simulink library "lib_wheel2"  (Simulink 10.1)
settings: Solver=VariableStepAuto  StartTime=0.0  StopTime=10.0  RelTol=1e-3
undefined symbols (not defined in the file or in its folder): lib_help, NOTES, veh_air_density, veh_CD, veh_cg_height, veh_FA, veh_front_wt_frac, veh_gravity, veh_roadwheel_radius, veh_rr_a, veh_rr_alpha, veh_rr_b, veh_rr_beta, veh_rr_c, veh_wheelbase, wh_1st_rrc, wh_2nd_rrc, wh_axle_loss_mass, wh_axle_loss_trq, wh_fa_dl_brake_frac, wh_fa_dl_brake_mph, wh_fa_fric_brake_frac, wh_fa_fric_brake_mph, wh_front_active_bool, wh_inertia, wh_max_front_brake_force, wh_max_rear_brake_force, wh_pressure, wh_radius, wh_rear_active_bool, wh_slip, wh_slip_force_coeff
undefined symbols (not defined in the file): logFlag
libraries: $bdroot x61, lib_vehicle x2, lib_etc x2, lib_controls x2, lib_wheel x1
(part 2 of 13)

== system lib_wheel2/Submodels/front and rear brake controller (achievable)/braking force supplied by front friction brakes (N) ==
  add'l braking force req'd (N) : Inport
  possible speed (mph) : Inport  Port=2
  max front brake force (N) : Inport  Port=3
  Block NOTES : Subsystem
      mask Display: disp('Block\nNOTES')
  Constant : Constant  Value=1+eps
  Constant1 : Constant  Value=0.6
  Keep 0<frac<1 : Saturate  UpperLimit=1  LowerLimit=0
  MinMax : MinMax  Function=max  Inputs=2
  Product : Product  Inputs=**  SaturateOnIntegerOverflow=on
  Product1 : Product  Inputs=*/  SaturateOnIntegerOverflow=on
  Saturation : Saturate  UpperLimit=max(wh_fa_fric_brake_mph)  LowerLimit=min(wh_fa_fric_brake_mph)
  Saturation1 : Saturate  UpperLimit=max(wh_fa_dl_brake_mph)  LowerLimit=min(wh_fa_dl_brake_mph)
  Sum : Sum  Inputs=-+  SaturateOnIntegerOverflow=on
  Switch1 : Switch  Threshold=eps  SaturateOnIntegerOverflow=on  InputSameDT=on
  driveline braking fraction : Lookup  InputValues=wh_fa_dl_brake_mph  Table=wh_fa_dl_brake_frac  SaturateOnIntegerOverflow=on
  front friction braking fraction : Lookup  InputValues=wh_fa_fric_brake_mph  Table=wh_fa_fric_brake_frac  SaturateOnIntegerOverflow=on
  braking force from front-axle friction brakes (N) : Outport  InitialOutput=0
  wires:
  Keep 0<frac<1/1 -> Product/2
  Switch1/1 -> Keep 0<frac<1/1
  MinMax/1 -> braking force from front-axle friction brakes (N)/1
  Product/1 -> MinMax/1
  max front brake force (N)/1 -> MinMax/2
  add'l braking force req'd (N)/1 -> Product/1
  Constant/1 -> Sum/2
  driveline braking fraction/1 -> Sum/1
  front friction braking fraction/1 -> Product1/1
  Product1/1 -> Switch1/1
  Sum/1 -> Product1/2, Switch1/2
  Constant1/1 -> Switch1/3
  Saturation/1 -> front friction braking fraction/1
  Saturation1/1 -> driveline braking fraction/1
  possible speed (mph)/1 -> Saturation1/1, Saturation/1

== system lib_wheel2/Submodels/traction control 2 axle/Block NOTES ==
  note: Requested speed and force are limited by the
      | tractive characteristics of the tires in this block.

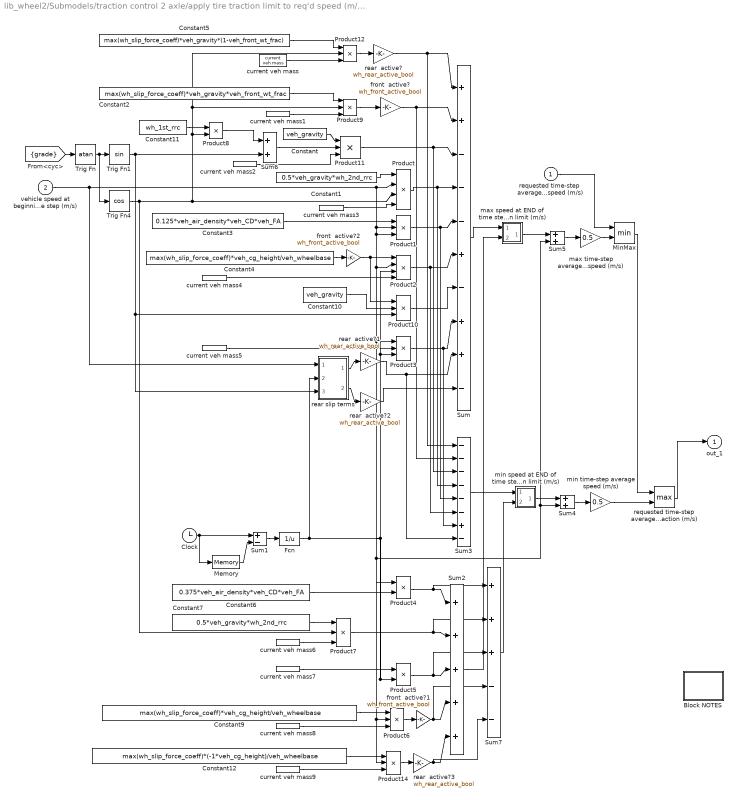
== system lib_wheel2/Submodels/traction control 2 axle/apply tire traction limit to req'd speed (m/s) ==
  "requested time-step  average vehicle speed (m/s) " : Inport
  vehicle speed at beginning of time step (m/s) : Inport  Port=2
  Block NOTES : Subsystem
      mask Display: disp('Block\nNOTES')
  Clock : Clock
  Constant : Constant  Value=veh_gravity
  Constant1 : Constant  Value=0.5*veh_gravity*wh_2nd_rrc
  Constant10 : Constant  Value=veh_gravity
  Constant11 : Constant  Value=wh_1st_rrc
  Constant12 : Constant  Value=max(wh_slip_force_coeff)*(-1*veh_cg_height)/veh_wheelbase
  Constant2 : Constant  Value=max(wh_slip_force_coeff)*veh_gravity*veh_front_wt_frac
  Constant3 : Constant  Value=0.125*veh_air_density*veh_CD*veh_FA
  Constant4 : Constant  Value=max(wh_slip_force_coeff)*veh_cg_height/veh_wheelbase
  Constant5 : Constant  Value=max(wh_slip_force_coeff)*veh_gravity*(1-veh_front_wt_frac)
  Constant6 : Constant  Value=0.375*veh_air_density*veh_CD*veh_FA
  Constant7 : Constant  Value=0.5*veh_gravity*wh_2nd_rrc
  Constant9 : Constant  Value=max(wh_slip_force_coeff)*veh_cg_height/veh_wheelbase
  Fcn : Fcn  Expr=1/u
  Memory : Memory  InitialCondition=-0.1
  MinMax : MinMax  Inputs=2
  Product : Product  Inputs=4  SaturateOnIntegerOverflow=on
  Product{1,3,6..7,9..12,14} (9 alike) : Product  Inputs=3  SaturateOnIntegerOverflow=on
  Product2 : Product  Inputs=4  SaturateOnIntegerOverflow=on
  Product4 : Product  SaturateOnIntegerOverflow=on
  Product5 : Product  SaturateOnIntegerOverflow=on
  Product8 : Product  SaturateOnIntegerOverflow=on
  Sum : Sum  Inputs=++---+-++-  SaturateOnIntegerOverflow=on
  Sum1 : Sum  Inputs=+-  SaturateOnIntegerOverflow=on
  Sum2 : Sum  Inputs=+++++  SaturateOnIntegerOverflow=on
  Sum3 : Sum  Inputs=------+-  SaturateOnIntegerOverflow=on
  Sum4 : Sum  SaturateOnIntegerOverflow=on
  Sum5 : Sum  SaturateOnIntegerOverflow=on
  Sum6 : Sum  SaturateOnIntegerOverflow=on
  Sum7 : Sum  Inputs=+++--  SaturateOnIntegerOverflow=on
  Trig Fn4 : Trigonometry  Operator=cos
  Trig Fn : Trigonometry  Operator=atan
  Trig Fn1 : Trigonometry
  current veh mass{,1..9} (10 alike) : $bdroot/Submodels/current veh mass
      settings: RTWFcnNameOpts=Auto  RTWFileNameOpts=Auto
  front  active? : Gain  Gain=wh_front_active_bool  SaturateOnIntegerOverflow=on
  front  active?1 : Gain  Gain=wh_front_active_bool  SaturateOnIntegerOverflow=on
  front  active?2 : Gain  Gain=wh_front_active_bool  SaturateOnIntegerOverflow=on
  max speed at END of time step given tire traction limit (m/s) : Subsystem
      mask Display: disp('/')
  max time-step average speed (m/s) : Gain  Gain=0.5  SaturateOnIntegerOverflow=on
  min speed at END of time step given tire traction limit (m/s) : Subsystem
      mask Display: disp('/')
  min time-step average speed (m/s) : Gain  Gain=0.5  SaturateOnIntegerOverflow=on
  rear  active?{,1..3} (4 alike) : Gain  Gain=wh_rear_active_bool  SaturateOnIntegerOverflow=on
  rear slip terms : Subsystem
  requested time-step average speed limited by tire traction (m/s) : MinMax  Function=max  Inputs=2
  out_1 : Outport  InitialOutput=0
  wires:
  Constant1/1 -> Product/1
  Constant3/1 -> Product1/1
  Fcn/1 -> Product2/3, Product3/3, Product5/2, Product6/2, Product14/2, rear slip terms/2(1/dt)
  Sum/1 -> max speed at END of time step given tire traction limit (m/s)/1(in_1)
  Product1/1 -> Sum/5, Sum3/5
  Product/1 -> Sum/4, Sum3/4
  Product9/1 -> front  active?/1
  Product2/1 -> Sum/6, Sum3/6
  max speed at END of time step given tire traction limit (m/s)/1(out_1) -> Sum5/1
  [grade] -> Trig Fn/1
  vehicle speed at beginning of time step (m/s)/1 -> Product/2, Product1/2, Product1/3, Product2/2, Product3/1, Product4/1, Sum4/2, Sum5/2, rear slip terms/1(initial speed)
  Trig Fn/1 -> Trig Fn1/1, Trig Fn4/1
  Product6/1 -> front  active?1/1
  Product5/1 -> Sum7/3, Sum2/3
  Product7/1 -> Sum7/2, Sum2/2
  Product4/1 -> Sum7/1, Sum2/1
  Constant6/1 -> Product4/2
  Constant9/1 -> Product6/1
  Constant7/1 -> Product7/1
  Sum7/1 -> min speed at END of time step given tire traction limit (m/s)/2(in_2)
  Sum3/1 -> min speed at END of time step given tire traction limit (m/s)/1(in_1)
  MinMax/1 -> requested time-step average speed limited by tire traction (m/s)/1
  min speed at END of time step given tire traction limit (m/s)/1(out_1) -> Sum4/1
  Sum4/1 -> min time-step average speed (m/s)/1
  requested time-step average speed limited by tire traction (m/s)/1 -> out_1/1
  min time-step average speed (m/s)/1 -> requested time-step average speed limited by tire traction (m/s)/2
  Sum2/1 -> max speed at END of time step given tire traction limit (m/s)/2(in_2)
  current veh mass7/1 -> Product5/1
  Memory/1 -> Sum1/2
  Sum1/1 -> Fcn/1
  Clock/1 -> Sum1/1, Memory/1
  Trig Fn4/1 -> Product7/2, Product/3, Product8/2, Product9/2, Product12/2
  Product8/1 -> Sum6/1
  Constant11/1 -> Product8/1
  Constant2/1 -> Product9/1
  Sum5/1 -> max time-step average speed (m/s)/1
  "requested time-step  average vehicle speed (m/s) "/1 -> MinMax/1
  max time-step average speed (m/s)/1 -> MinMax/2
  current veh mass5/1 -> Product3/2
  Product3/1 -> Sum/8, Sum3/7
  Product10/1 -> Sum/7
  Constant4/1 -> front  active?2/1
  Constant10/1 -> Product10/2
  Trig Fn1/1 -> Sum6/2, Product10/3, rear slip terms/3(sin(theta))
  Sum6/1 -> Product11/2
  Product11/1 -> Sum/3, Sum3/3
  Constant/1 -> Product11/1
  current veh mass2/1 -> Product11/3
  current veh mass3/1 -> Product/4
  current veh mass1/1 -> Product9/3
  current veh mass4/1 -> Product2/4
  current veh mass6/1 -> Product7/3
  current veh mass8/1 -> Product6/3
  Product12/1 -> rear  active?/1
  Constant5/1 -> Product12/1
  current veh mass/1 -> Product12/3
  rear  active?/1 -> Sum/1, Sum3/1
  rear slip terms/1(Out1) -> rear  active?1/1
  rear slip terms/2(Out2) -> rear  active?2/1
  Product14/1 -> rear  active?3/1
  Constant12/1 -> Product14/1
  current veh mass9/1 -> Product14/3
  rear  active?1/1 -> Sum/9, Sum3/8
  rear  active?2/1 -> Sum/10
  rear  active?3/1 -> Sum7/5, Sum2/5
  front  active?/1 -> Sum/2, Sum3/2
  front  active?1/1 -> Sum7/4, Sum2/4
  front  active?2/1 -> Product2/1, Product10/1

== system lib_wheel2/Submodels/traction control 2 axle/enforce max.  front axle tractive force  due to slip (N) ==
  tractive force req'd at tire/road interface (N) : Inport
  requested time-step average vehicle speed (m/s) : Inport  Port=2
  speed at beginning of time step (m/s) : Inport  Port=3
  " " : MinMax  Inputs=2
  Block NOTES : Subsystem
      mask Display: disp('Block\nNOTES')
  Constant2 : Constant  Value=max(wh_slip_force_coeff)
  Gain : Gain  Gain=-1  SaturateOnIntegerOverflow=on
  Product1 : Product  SaturateOnIntegerOverflow=on
  Product2 : Product  SaturateOnIntegerOverflow=on
  Product3 : Product  Inputs=*/  SaturateOnIntegerOverflow=on
  Product4 : Product  Inputs=*/  SaturateOnIntegerOverflow=on
  Sum1 : Sum  SaturateOnIntegerOverflow=on
  Sum2 : Sum  SaturateOnIntegerOverflow=on
  front : Subsystem
  front  active? : Gain  Gain=wh_front_active_bool  SaturateOnIntegerOverflow=on
  front traction ratio : ToWorkspace  VariableName=front_traction_ratio_orig
  rear : Subsystem
  rear  active? : Gain  Gain=wh_rear_active_bool  SaturateOnIntegerOverflow=on
  tractive force request limited by slip-threshhold force (N)1 : MinMax  Function=max  Inputs=2
  slip-limited force (N) : Outport  InitialOutput=0
  weight on front axle (N) : Outport  Port=2  InitialOutput=0
  weight on rear axle (N) : Outport  Port=3  InitialOutput=0
  front/total traction ratio : Outport  Port=4  InitialOutput=0
  wires:
  front/1(Out1) -> Product2/1, weight on front axle (N)/1
  requested time-step average vehicle speed (m/s)/1 -> front/1(In1), rear/1(In1)
  speed at beginning of time step (m/s)/1 -> front/2(In2), rear/2(In2)
  Gain/1 -> tractive force request limited by slip-threshhold force (N)1/2
  Constant2/1 -> Product2/2, Product1/2
  tractive force req'd at tire/road interface (N)/1 -> " "/2
  " "/1 -> tractive force request limited by slip-threshhold force (N)1/1
  tractive force request limited by slip-threshhold force (N)1/1 -> slip-limited force (N)/1
  rear/1(Out1) -> weight on rear axle (N)/1, Product1/1
  Sum1/1 -> " "/1, Gain/1, Product3/2
  Product1/1 -> rear  active?/1, Sum2/2
  Product2/1 -> front  active?/1, Sum2/1, Product4/1
  Product3/1 -> front/total traction ratio/1
  front  active?/1 -> Sum1/1, Product3/1
  rear  active?/1 -> Sum1/2
  Sum2/1 -> Product4/2
  Product4/1 -> front traction ratio/1

== system lib_wheel2/Submodels/traction control J2452 2 axle/Block NOTES ==
  note: Requested speed and force are limited by the
      | tractive characteristics of the tires in this block.

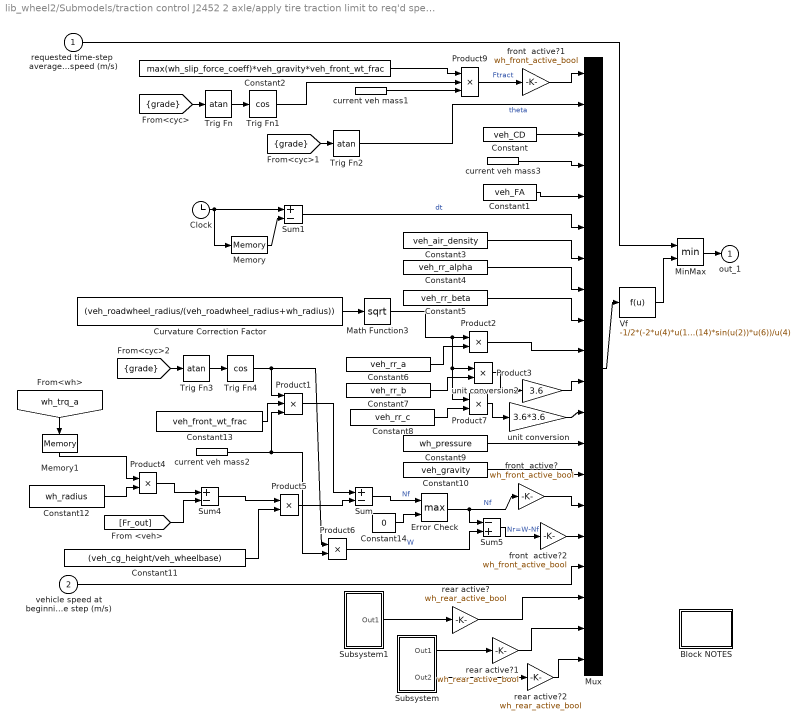
== system lib_wheel2/Submodels/traction control J2452 2 axle/apply tire traction limit to req'd speed (m/s) ==
  "requested time-step  average vehicle speed (m/s) " : Inport
  vehicle speed at beginning of time step (m/s) : Inport  Port=2
  Block NOTES : Subsystem
      mask Display: disp('Block\nNOTES')
  Clock : Clock
  Constant : Constant  Value=veh_CD
  Constant1 : Constant  Value=veh_FA
  Constant10 : Constant  Value=veh_gravity
  Constant11 : Constant  Value=(veh_cg_height/veh_wheelbase)
  Constant12 : Constant  Value=wh_radius
  Constant13 : Constant  Value=veh_front_wt_frac
  Constant14 : Constant  Value=0
  Constant2 : Constant  Value=max(wh_slip_force_coeff)*veh_gravity*veh_front_wt_frac
  Constant3 : Constant  Value=veh_air_density
  Constant4 : Constant  Value=veh_rr_alpha
  Constant5 : Constant  Value=veh_rr_beta
  Constant6 : Constant  Value=veh_rr_a
  Constant7 : Constant  Value=veh_rr_b
  Constant8 : Constant  Value=veh_rr_c
  Constant9 : Constant  Value=wh_pressure
  Curvature Correction Factor : Constant  Value=(veh_roadwheel_radius/(veh_roadwheel_radius+wh_radius))  VectorParams1D=off
  Error Check : MinMax  Function=max  Inputs=2
  Math Function3 : Math  Operator=sqrt  SaturateOnIntegerOverflow=on
  Memory : Memory  InitialCondition=-0.1
  Memory1 : Memory  InitialCondition=-0.1
  MinMax : MinMax  Inputs=2
  Mux : Mux  Inputs=20
  Product1 : Product  Inputs=3  SaturateOnIntegerOverflow=on
  Product{2..7} (6 alike) : Product  SaturateOnIntegerOverflow=on
  Product9 : Product  Inputs=3  SaturateOnIntegerOverflow=on
  Subsystem : Subsystem
  Subsystem1 : Subsystem
  Sum : Sum  Inputs=+-  SaturateOnIntegerOverflow=on
  Sum1 : Sum  Inputs=+-  SaturateOnIntegerOverflow=on
  Sum4 : Sum  Inputs=+-  SaturateOnIntegerOverflow=on
  Sum5 : Sum  Inputs=-+  SaturateOnIntegerOverflow=on
  Trig Fn : Trigonometry  Operator=atan
  Trig Fn1 : Trigonometry  Operator=cos
  Trig Fn2 : Trigonometry  Operator=atan
  Trig Fn3 : Trigonometry  Operator=atan
  Trig Fn4 : Trigonometry  Operator=cos
  Vf : Fcn  Expr=-1/2*(-2*u(4)*u(17)-2*u(1)*u(6)-2*u(18)*u(6)+4*u(13)^u(8)*u(6)*(1/2*u(15))^u(9)*u(10)+4*u(13)^u(8)*u(6)*(1/2*u(19))^u(9)*u(10)+4*u(13)^u(8)*u(6)*(1/2*u(15))^u(9)*u(11)*u(17)+4*u(13)^u(8)*u(6)*(1/2*u(19))^u(9)*u(11)*u(17)+4*u(13)^u(8)*u(6)*(1/2*u(15))^u(9)*u(12)*u(17)^2+4*u(13)^u(8)*u(6)*(1/2*u(19))^u(9)*u(12)*u(17)^2+4*u(13)^u(8)*u(6)*(1/2*u(16))^u(9)*u(10)+4*u(13)^u(8)*u(6)*(1/2*u(20))^u(9)*u(10)+4*u(13)^u(8)*u(6)*(1/2*u(16))^u(9)*u(11)*u(17)+4*u(13)^u(8)*u(6)*(1/2*u(20))^u(9)*u(11)*u(17)+4*u(13)^u(8)*u(6)*(1/2*u(16))^u(9)*u(12)*u(17)^2+4*u(13)^u(8)*u(6)*(1/2*u(20))^u(9)*u(12)*u(17)^2+u(7)*u(3)*u(5)*u(17)^2*u(6)+2*u(4)*u(14)*sin(u(2))*u(6))/u(4)
  current veh mass1 : $bdroot/Submodels/current veh mass
      settings: RTWFcnNameOpts=Auto  RTWFileNameOpts=Auto
  current veh mass2 : $bdroot/Submodels/current veh mass
      settings: RTWFcnNameOpts=Auto  RTWFileNameOpts=Auto
  current veh mass3 : $bdroot/Submodels/current veh mass
      settings: RTWFcnNameOpts=Auto  RTWFileNameOpts=Auto
  front  active? : Gain  Gain=wh_front_active_bool  SaturateOnIntegerOverflow=on
  front  active?1 : Gain  Gain=wh_front_active_bool  SaturateOnIntegerOverflow=on
  front  active?2 : Gain  Gain=wh_front_active_bool  SaturateOnIntegerOverflow=on
  rear active? : Gain  Gain=wh_rear_active_bool  SaturateOnIntegerOverflow=on
  rear active?1 : Gain  Gain=wh_rear_active_bool  SaturateOnIntegerOverflow=on
  rear active?2 : Gain  Gain=wh_rear_active_bool  SaturateOnIntegerOverflow=on
  unit conversion : Gain  Gain=3.6*3.6  SaturateOnIntegerOverflow=on
  unit conversion2 : Gain  Gain=3.6  SaturateOnIntegerOverflow=on
  out_1 : Outport  InitialOutput=0
  wires:
  Product7/1 -> unit conversion/1
  Constant8/1 -> Product7/2
  Product3/1 -> unit conversion2/1
  Constant7/1 -> Product3/2
  Product2/1 -> Mux/10
  Constant6/1 -> Product2/2
  Math Function3/1 -> Product7/1, Product3/1, Product2/1
  Curvature Correction Factor/1 -> Math Function3/1
  unit conversion/1 -> Mux/12
  unit conversion2/1 -> Mux/11
  Error Check/1 -> Sum5/1, front  active?/1  "Nf"
  Constant14/1 -> Error Check/2
  Sum/1 -> Error Check/1  "Nf"
  Sum5/1 -> front  active?2/1  "Nr=W-Nf"
  Product6/1 -> Sum5/2  "W"
  Memory1/1 -> Product4/1
  [wh_trq_a] -> Memory1/1
  vehicle speed at beginning of time step (m/s)/1 -> Mux/17
  current veh mass2/1 -> Product6/2, Product1/3
  Constant13/1 -> Product1/2
  Trig Fn4/1 -> Product6/1, Product1/1
  Trig Fn3/1 -> Trig Fn4/1
  [grade] -> Trig Fn3/1
  Constant10/1 -> Mux/14
  Constant9/1 -> Mux/13
  Constant5/1 -> Mux/9
  Constant4/1 -> Mux/8
  Constant3/1 -> Mux/7
  Constant1/1 -> Mux/5
  current veh mass3/1 -> Mux/4
  Constant/1 -> Mux/3
  Mux/1 -> Vf/1
  Trig Fn1/1 -> Product9/2
  current veh mass1/1 -> Product9/3
  "requested time-step  average vehicle speed (m/s) "/1 -> MinMax/1
  Constant2/1 -> Product9/1
  Trig Fn/1 -> Trig Fn1/1
  [grade] -> Trig Fn/1
  Product9/1 -> front  active?1/1  "Ftract"
  Sum1/1 -> Mux/6  "dt"
  Clock/1 -> Memory/1, Sum1/1
  Memory/1 -> Sum1/2
  [grade] -> Trig Fn2/1
  Trig Fn2/1 -> Mux/2  "theta"
  Product1/1 -> Sum/1
  MinMax/1 -> out_1/1
  Constant12/1 -> Product4/2
  Product4/1 -> Sum4/1
  [Fr_out] -> Sum4/2
  Sum4/1 -> Product5/1
  Constant11/1 -> Product5/2
  Product5/1 -> Sum/2
  Vf/1 -> MinMax/2
  Subsystem1/1(Out1) -> rear active?/1
  Subsystem/1(Out1) -> rear active?1/1
  Subsystem/2(Out2) -> rear active?2/1
  front  active?1/1 -> Mux/1
  front  active?/1 -> Mux/15
  front  active?2/1 -> Mux/16
  rear active?/1 -> Mux/18
  rear active?2/1 -> Mux/20
  rear active?1/1 -> Mux/19

== system lib_wheel2/Submodels/vehicle speed (m/s)/Block NOTES ==
  note: The actual vehicle speed at the end of the time step is taken as
      | the LESSER of the speed computed from the actual force and the speed
      | computed from the actual drivetrain speed if the required acceleration
      |  is greater than -1 m/s^2.  Otherwise, the GREATER of the two values is used.
      | Thus the worse acceleration rate is allowed if the vehicle is accelerating,
      | and the worse deceleration rate is allowed if the vehicle is decelerating.
      |
      | In no case will the computed speed fall below zero.
  note: Given the tractive force available, this block uses straightforward vehicle
      | dynamics equations to determine the achievable speed.

== system lib_wheel2/Submodels/vehicle speed (m/s)/b ==
  dt : Inport
  angle of elevation : Inport  Port=2
  vehicle moving? : Inport  Port=3
  Constant9 : Constant  Value=veh_gravity*wh_2nd_rrc
  Gain : Gain  Gain=2  SaturateOnIntegerOverflow=on
  Product10 : Product  Inputs=4  SaturateOnIntegerOverflow=on
  Product6 : Product  Inputs=*/  SaturateOnIntegerOverflow=on
  Sum : Sum  SaturateOnIntegerOverflow=on
  Trig Fn7 : Trigonometry  Operator=cos
  current veh mass1 : $bdroot/Submodels/current veh mass
      settings: RTWFcnNameOpts=Auto  RTWFileNameOpts=Auto
  current veh mass2 : $bdroot/Submodels/current veh mass
      settings: RTWFcnNameOpts=Auto  RTWFileNameOpts=Auto
  b : Outport
  wires:
  current veh mass2/1 -> Product10/4
  current veh mass1/1 -> Gain/1
  vehicle moving?/1 -> Product10/3
  angle of elevation/1 -> Trig Fn7/1
  dt/1 -> Product6/2
  Sum/1 -> b/1
  Product10/1 -> Sum/2
  Constant9/1 -> Product10/1
  Trig Fn7/1 -> Product10/2
  Product6/1 -> Sum/1
  Gain/1 -> Product6/1

== system lib_wheel2/Submodels/vehicle speed (m/s)/c ==
  dt : Inport
  v_prev : Inport  Port=2
  Ftract : Inport  Port=3
  angle of elevation : Inport  Port=4
  vehicle moving? : Inport  Port=5
  Constant1 : Constant  Value=inf
  Constant12 : Constant  Value=wh_1st_rrc
  Constant13 : Constant  Value=veh_gravity
  Constant2 : Constant  Value=-70
  Gain : Gain  Gain=2  SaturateOnIntegerOverflow=on
  Product1 : Product  Inputs=**  SaturateOnIntegerOverflow=on
  Product7 : Product  Inputs=*/*  SaturateOnIntegerOverflow=on
  Product8 : Product  Inputs=3  SaturateOnIntegerOverflow=on
  Product9 : Product  Inputs=3  SaturateOnIntegerOverflow=on
  Sum : Sum  Inputs=--+  SaturateOnIntegerOverflow=on
  Sum6 : Sum  SaturateOnIntegerOverflow=on
  Trig Fn : Trigonometry  Operator=cos
  Trig Fn2 : Trigonometry
  current veh mass : $bdroot/Submodels/current veh mass
      settings: RTWFcnNameOpts=Auto  RTWFileNameOpts=Auto
  current veh mass1 : $bdroot/Submodels/current veh mass
      settings: RTWFcnNameOpts=Auto  RTWFileNameOpts=Auto
  current veh mass2 : $bdroot/Submodels/current veh mass
      settings: RTWFcnNameOpts=Auto  RTWFileNameOpts=Auto
  saturation with inputs : lib_etc/saturation with inputs
      settings: RTWFcnNameOpts=Auto  RTWFileNameOpts=Auto
  c : Outport
  wires:
  current veh mass2/1 -> Product8/3
  current veh mass1/1 -> Gain/1
  Gain/1 -> Product7/1
  dt/1 -> Product7/2
  Sum/1 -> c/1
  Product8/1 -> Sum/3
  Constant13/1 -> Product8/2
  Sum6/1 -> Product8/1
  vehicle moving?/1 -> Product9/3
  Trig Fn2/1 -> Sum6/2
  angle of elevation/1 -> Trig Fn2/1, Trig Fn/1
  Product9/1 -> Sum6/1
  Trig Fn/1 -> Product9/2
  Constant12/1 -> Product9/1
  Ftract/1 -> saturation with inputs/2
  saturation with inputs/1 -> Sum/2
  Product7/1 -> Sum/1
  v_prev/1 -> Product7/3
  Constant2/1 -> Product1/2
  Constant1/1 -> saturation with inputs/1
  current veh mass/1 -> Product1/1
  Product1/1 -> saturation with inputs/3

== system lib_wheel2/Submodels/vehicle speed (m/s) j2452/Block NOTES ==
  note: Rolling resistance force was brought into model to solve the quadratic.
      | Veh_rr_b and veh_rr_c were converted to the proper units.
  note: Given the tractive force available, this block uses straightforward vehicle
      | dynamics equations to determine the achievable speed.
  note: The actual vehicle speed at the end of the time step is taken as
      | the LESSER of the speed computed from the actual force and the speed
      | computed from the actual drivetrain speed if the required acceleration
      |  is greater than -1 m/s^2.  Otherwise, the GREATER of the two values is used.
      | Thus the worse acceleration rate is allowed if the vehicle is accelerating,
      | and the worse deceleration rate is allowed if the vehicle is decelerating.
      |
      | In no case will the computed speed fall below zero.

== system lib_wheel2/Submodels/vehicle speed (m/s) j2452/b ==
  dt : Inport
  angle of elevation : Inport  Port=2
  vehicle moving? : Inport  Port=3
  Constant1 : Constant  Value=wh_pressure^veh_rr_alpha  VectorParams1D=off
  Constant13 : Constant  Value=veh_gravity
  Constant9 : Constant  Value=veh_rr_b  VectorParams1D=off
  Curvature Correction Factor : Constant  Value=(veh_roadwheel_radius/(veh_roadwheel_radius+wh_radius))  VectorParams1D=off
  Gain : Gain  Gain=2  SaturateOnIntegerOverflow=on
  Math Function : Math  Operator=pow  SaturateOnIntegerOverflow=on
  Math Function3 : Math  Operator=sqrt  SaturateOnIntegerOverflow=on
  Product1 : Product  Inputs=4  SaturateOnIntegerOverflow=on
  Product10 : Product  Inputs=3  SaturateOnIntegerOverflow=on
  Product2 : Product  SaturateOnIntegerOverflow=on
  Product6 : Product  Inputs=*/  SaturateOnIntegerOverflow=on
  Sum : Sum  SaturateOnIntegerOverflow=on
  Trig Fn7 : Trigonometry  Operator=cos
  beta : Constant  Value=veh_rr_beta
  current veh mass1 : $bdroot/Submodels/current veh mass
      settings: RTWFcnNameOpts=Auto  RTWFileNameOpts=Auto
  current veh mass2 : $bdroot/Submodels/current veh mass
      settings: RTWFcnNameOpts=Auto  RTWFileNameOpts=Auto
  unit conversion N/km/h to N/m/s : Gain  Gain=3.6  SaturateOnIntegerOverflow=on
  b : Outport
  wires:
  Product2/1 -> Product1/1
  Math Function3/1 -> Product2/2
  unit conversion N/km/h to N/m/s/1 -> Product2/1
  Curvature Correction Factor/1 -> Math Function3/1
  Constant13/1 -> Product10/3
  Product1/1 -> Sum/2
  vehicle moving?/1 -> Product1/4
  Constant1/1 -> Product1/3
  Math Function/1 -> Product1/2
  Constant9/1 -> unit conversion N/km/h to N/m/s/1
  beta/1 -> Math Function/2
  Product10/1 -> Math Function/1
  current veh mass2/1 -> Product10/2
  Trig Fn7/1 -> Product10/1
  Gain/1 -> Product6/1
  Product6/1 -> Sum/1
  Sum/1 -> b/1
  dt/1 -> Product6/2
  angle of elevation/1 -> Trig Fn7/1
  current veh mass1/1 -> Gain/1

== system lib_wheel2/Submodels/vehicle speed (m/s) j2452/c ==
  dt : Inport
  v_prev : Inport  Port=2
  Ftract : Inport  Port=3
  angle of elevation : Inport  Port=4
  vehicle moving? : Inport  Port=5
  Constant1 : Constant  Value=inf
  Constant13 : Constant  Value=veh_gravity
  Constant2 : Constant  Value=-70
  Curvature Correction Factor : Constant  Value=(veh_roadwheel_radius/(veh_roadwheel_radius+wh_radius))  VectorParams1D=off
  Gain : Gain  Gain=2  SaturateOnIntegerOverflow=on
  Math Function : Math  Operator=pow  SaturateOnIntegerOverflow=on
  Math Function3 : Math  Operator=sqrt  SaturateOnIntegerOverflow=on
  Product1 : Product  Inputs=**  SaturateOnIntegerOverflow=on
  Product7 : Product  Inputs=*/*  SaturateOnIntegerOverflow=on
  Product8 : Product  Inputs=5  SaturateOnIntegerOverflow=on
  Product9 : Product  Inputs=3  SaturateOnIntegerOverflow=on
  Sum : Sum  Inputs=--+  SaturateOnIntegerOverflow=on
  Trig Fn : Trigonometry  Operator=cos
  a : Constant  Value=veh_rr_a
  alpha : Constant  Value=wh_pressure^veh_rr_alpha
  beta : Constant  Value=veh_rr_beta
  current veh mass : $bdroot/Submodels/current veh mass
      settings: RTWFcnNameOpts=Auto  RTWFileNameOpts=Auto
  current veh mass1 : $bdroot/Submodels/current veh mass
      settings: RTWFcnNameOpts=Auto  RTWFileNameOpts=Auto
  current veh mass2 : $bdroot/Submodels/current veh mass
      settings: RTWFcnNameOpts=Auto  RTWFileNameOpts=Auto
  saturation with inputs : lib_etc/saturation with inputs
      settings: RTWFcnNameOpts=Auto  RTWFileNameOpts=Auto
  c : Outport
  wires:
  vehicle moving?/1 -> Product8/5
  Math Function3/1 -> Product8/4
  Curvature Correction Factor/1 -> Math Function3/1
  a/1 -> Product8/3
  alpha/1 -> Product8/2
  Math Function/1 -> Product8/1
  beta/1 -> Math Function/2
  Product9/1 -> Math Function/1
  Trig Fn/1 -> Product9/3
  current veh mass2/1 -> Product9/2
  Constant13/1 -> Product9/1
  v_prev/1 -> Product7/3
  Product7/1 -> Sum/1
  saturation with inputs/1 -> Sum/2
  Ftract/1 -> saturation with inputs/2
  angle of elevation/1 -> Trig Fn/1
  Product8/1 -> Sum/3
  Sum/1 -> c/1
  dt/1 -> Product7/2
  Gain/1 -> Product7/1
  current veh mass1/1 -> Gain/1
  Constant2/1 -> Product1/2
  Constant1/1 -> saturation with inputs/1
  current veh mass/1 -> Product1/1
  Product1/1 -> saturation with inputs/3

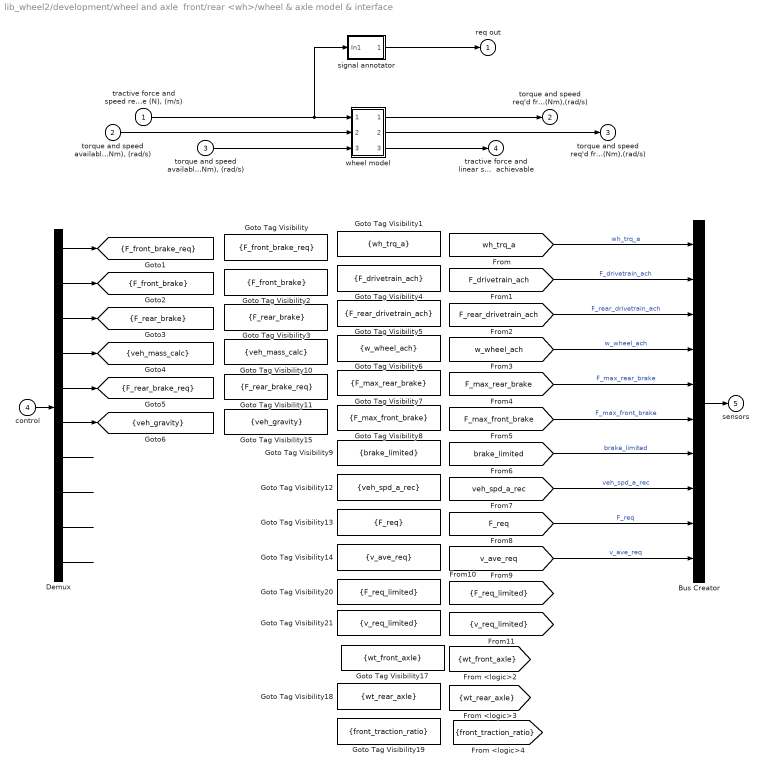
== system lib_wheel2/development/wheel and axle  front/rear <wh>/wheel & axle model & interface ==
  "tractive force and speed req'd of tire/road interface (N), (m/s)" : Inport
  "torque and speed available from drivetrain into front axle (Nm), (rad/s)" : Inport  Port=2
  "torque and speed available from drivetrain into rear axle (Nm), (rad/s)" : Inport  Port=3
  control : Inport  Port=4
  Bus Creator : BusCreator  Inputs=10
  Demux : Demux  Outputs=10
  Goto Tag Visibility : GotoTagVisibility  GotoTag=F_front_brake_req
  Goto Tag Visibility1 : GotoTagVisibility  GotoTag=wh_trq_a
  Goto Tag Visibility10 : GotoTagVisibility  GotoTag=veh_mass_calc
  Goto Tag Visibility11 : GotoTagVisibility  GotoTag=F_rear_brake_req
  Goto Tag Visibility12 : GotoTagVisibility  GotoTag=veh_spd_a_rec
  Goto Tag Visibility13 : GotoTagVisibility  GotoTag=F_req
  Goto Tag Visibility14 : GotoTagVisibility  GotoTag=v_ave_req
  Goto Tag Visibility15 : GotoTagVisibility  GotoTag=veh_gravity
  Goto Tag Visibility17 : GotoTagVisibility  GotoTag=wt_front_axle
  Goto Tag Visibility18 : GotoTagVisibility  GotoTag=wt_rear_axle
  Goto Tag Visibility19 : GotoTagVisibility  GotoTag=front_traction_ratio
  Goto Tag Visibility2 : GotoTagVisibility  GotoTag=F_front_brake
  Goto Tag Visibility20 : GotoTagVisibility  GotoTag=F_req_limited
  Goto Tag Visibility21 : GotoTagVisibility  GotoTag=v_req_limited
  Goto Tag Visibility3 : GotoTagVisibility  GotoTag=F_rear_brake
  Goto Tag Visibility4 : GotoTagVisibility  GotoTag=F_drivetrain_ach
  Goto Tag Visibility5 : GotoTagVisibility  GotoTag=F_rear_drivetrain_ach
  Goto Tag Visibility6 : GotoTagVisibility  GotoTag=w_wheel_ach
  Goto Tag Visibility7 : GotoTagVisibility  GotoTag=F_max_rear_brake
  Goto Tag Visibility8 : GotoTagVisibility  GotoTag=F_max_front_brake
  Goto Tag Visibility9 : GotoTagVisibility  GotoTag=brake_limited
  signal annotator : Subsystem
  wheel model : Subsystem
  req out : Outport  InitialOutput=0
  torque and speed req'd from drivetrain into front axle (Nm),(rad/s) : Outport  Port=2  InitialOutput=0
  torque and speed req'd from drivetrain into rear axle (Nm),(rad/s) : Outport  Port=3  InitialOutput=0
  tractive force and linear speed  achievable : Outport  Port=4  InitialOutput=0
  sensors : Outport  Port=5  InitialOutput=0
  tag scope: F_front_brake=scoped, F_front_brake_req=scoped, F_rear_brake=scoped, F_rear_brake_req=scoped, veh_gravity=scoped, veh_mass_calc=scoped
  wires:
  wheel model/1(torque and speed req'd from drivetrain into front axle (Nm),(rad/s)) -> torque and speed req'd from drivetrain into front axle (Nm),(rad/s)/1
  "tractive force and speed req'd of tire/road interface (N), (m/s)"/1 -> wheel model/1("tractive force and speed req'd of tire/road interface (N), (m/s)"), signal annotator/1(In1)
  wheel model/2(torque and speed req'd from drivetrain into rear axle (Nm),(rad/s)) -> torque and speed req'd from drivetrain into rear axle (Nm),(rad/s)/1
  "torque and speed available from drivetrain into front axle (Nm), (rad/s)"/1 -> wheel model/2("torque and speed available from drivetrain into front axle (Nm), (rad/s)")
  wheel model/3(tractive force and linear speed  achievable) -> tractive force and linear speed  achievable/1
  "torque and speed available from drivetrain into rear axle (Nm), (rad/s)"/1 -> wheel model/3("torque and speed available from drivetrain into rear axle (Nm), (rad/s)")
  signal annotator/1(Out1) -> req out/1
  control/1 -> Demux/1
  Demux/1 -> [F_front_brake_req]
  Demux/2 -> [F_front_brake]
  Demux/3 -> [F_rear_brake]
  Demux/4 -> [veh_mass_calc]
  Demux/5 -> [F_rear_brake_req]
  Demux/6 -> [veh_gravity]
  Demux/7 -> ?
  Demux/8 -> ?
  Demux/9 -> ?
  Demux/10 -> ?
  [wh_trq_a] -> Bus Creator/1  "wh_trq_a"
  [F_drivetrain_ach] -> Bus Creator/2  "F_drivetrain_ach"
  [F_rear_drivetrain_ach] -> Bus Creator/3  "F_rear_drivetrain_ach"
  [w_wheel_ach] -> Bus Creator/4  "w_wheel_ach"
  [F_max_rear_brake] -> Bus Creator/5  "F_max_rear_brake"
  [F_max_front_brake] -> Bus Creator/6  "F_max_front_brake"
  [brake_limited] -> Bus Creator/7  "brake_limited"
  [veh_spd_a_rec] -> Bus Creator/8  "veh_spd_a_rec"
  [F_req] -> Bus Creator/9  "F_req"
  [v_ave_req] -> Bus Creator/10  "v_ave_req"
  Bus Creator/1 -> sensors/1

== system lib_wheel2/development/wheel and axle  front/rear <wh> 2 axle --> 1 driveline/wheel & axle model & interface ==
  "tractive force and speed req'd of tire/road interface (N), (m/s)" : Inport
  "torque and speed available from drivetrain into axle (Nm), (rad/s)" : Inport  Port=2
  control : Inport  Port=3
  2 axle --> 1 driveline converter : Subsystem
  signal annotator : Subsystem
  wheel model : Subsystem
  req out : Outport  InitialOutput=0
  sensors : Outport  Port=2  InitialOutput=0
  tractive force and linear speed  achievable : Outport  Port=3  InitialOutput=0
  trq and spd into axle set required : Outport  Port=4  InitialOutput=0
  wires:
  wheel model/1(torque and speed req'd from drivetrain into front axle (Nm),(rad/s)) -> 2 axle --> 1 driveline converter/1(front req)
  "tractive force and speed req'd of tire/road interface (N), (m/s)"/1 -> wheel model/1("tractive force and speed req'd of tire/road interface (N), (m/s)"), signal annotator/1(In1)
  wheel model/2(torque and speed req'd from drivetrain into rear axle (Nm),(rad/s)) -> 2 axle --> 1 driveline converter/2(rear req)
  2 axle --> 1 driveline converter/2(front ach) -> wheel model/2("torque and speed available from drivetrain into front axle (Nm), (rad/s)")  "front axle"
  wheel model/3(tractive force and linear speed  achievable) -> tractive force and linear speed  achievable/1
  signal annotator/1(Out1) -> req out/1
  "torque and speed available from drivetrain into axle (Nm), (rad/s)"/1 -> 2 axle --> 1 driveline converter/3(ach)
  2 axle --> 1 driveline converter/3(rear ach) -> wheel model/3("torque and speed available from drivetrain into rear axle (Nm), (rad/s)")  "rear axle"
  2 axle --> 1 driveline converter/1(req) -> trq and spd into axle set required/1

== system lib_wheel2/vehicle, wheel, & axle front/rear <wh>/models and interface/slip, braking, traction calcs ==
  note: required force (N)
  note: Traction and Braking Calculations
  note: 4/-02-/2003, Michael O'Keefe
      |
      | Note: the goto tag "F_rear_brake_req" was added because it wasn't defined
      | anywhere else. Is this correct to define? Should it be defined elsewhere or as zero?
  Relational Operator : RelationalOperator  Operator=~=  RndMeth=Nearest  InputSameDT=on
  Sum : Sum  Inputs=-+  SaturateOnIntegerOverflow=on
  braking strategy : $bdroot/Submodels/braking strategy
      settings: RTWFcnNameOpts=Auto  RTWFileNameOpts=Auto
  config traction control : Subsystem  BlockChoice=traction control 2 axle
      settings: AttributesFormatString=%<BlockChoice>  TemplateBlock=lib_wheel2/Submodels/config traction control  MemberBlocks=traction control 2 axle,traction control J2452 2 axle
  front and rear brake controller (achievable) : $bdroot/Submodels/front and rear brake controller (achievable)
      settings: RTWFcnNameOpts=Auto  RTWFileNameOpts=Auto
  tag scope: F_front_brake=scoped, F_front_brake_req=scoped, F_rear_brake=scoped, F_rear_brake_req=scoped, F_req_limited=scoped, front_traction_ratio=scoped, slip_limited=scoped, v_req_limited=scoped, wt_front_axle=scoped, wt_rear_axle=scoped
  wires:
  front and rear brake controller (achievable)/1 -> [F_front_brake]
  [F_drivetrain_ach] -> front and rear brake controller (achievable)/2
  [w_wheel_ach] -> front and rear brake controller (achievable)/3
  [F_max_front_brake] -> front and rear brake controller (achievable)/4
  [F_max_rear_brake] -> front and rear brake controller (achievable)/5
  front and rear brake controller (achievable)/2 -> [F_rear_brake]
  [F_req] -> front and rear brake controller (achievable)/1
  braking strategy/2 -> Sum/1, [F_rear_brake_req]
  config traction control/1(req'd force (N)) -> Sum/2, Relational Operator/1, braking strategy/2
  braking strategy/1 -> [F_front_brake_req]
  [v_prev] -> config traction control/2(vehicle speed at beginning of time  step (m/s))
  config traction control/3(weight on front axle (N)) -> [wt_front_axle]
  [F_req] -> config traction control/3(total tractive force req'd (N))
  Sum/1 -> [F_req_limited]
  Relational Operator/1 -> [slip_limited]
  [F_req] -> Relational Operator/2
  [v_ave_req] -> config traction control/1(time-average vehicle speed  req'd (m/s))
  [v_ave_req] -> braking strategy/1
  config traction control/2(req'd speed (m/s)) -> [v_req_limited]
  config traction control/4(weight on rear axle (N)) -> [wt_rear_axle]
  config traction control/5(front/total  traction ratio) -> [front_traction_ratio]
  [F_rear_drivetrain_ach] -> front and rear brake controller (achievable)/6
